simulink model "diagrama_de_bloques"  (R2017b)
settings: Solver=FixedStepDiscrete  StartTime=0.0  StopTime=erle.T_simulacion  FixedStep=erle.Tm  RelTol=1e-3
undefined symbols (not defined in the file or in its folder): erle
settings Model: Creator=javi  LastModifiedBy=javi
settings DataIOCC: SaveFormat=Array

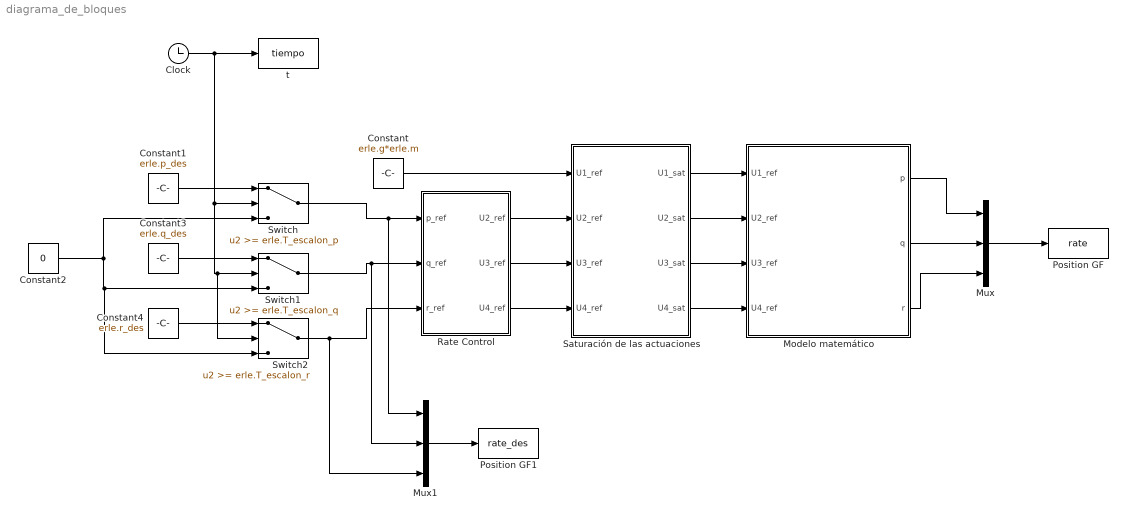
== system diagrama_de_bloques ==
  Clock : Clock
  Constant : Constant  Value=erle.g*erle.m
  Constant1 : Constant  Value=erle.p_des
  Constant2 : Constant  Value=0
  Constant3 : Constant  Value=erle.q_des
  Constant4 : Constant  Value=erle.r_des
  Modelo matemático : Subsystem
  Mux : Mux  Inputs=3
  Mux1 : Mux  Inputs=3
  Position GF : ToWorkspace  VariableName=rate  SampleTime=erle.Tm
  Position GF1 : ToWorkspace  VariableName=rate_des  SampleTime=erle.Tm
  Rate Control : Subsystem
  Saturación de las actuaciones : Subsystem
  Switch : Switch  Threshold=erle.T_escalon_p
  Switch1 : Switch  Threshold=erle.T_escalon_q
  Switch2 : Switch  Threshold=erle.T_escalon_r
  "t " : ToWorkspace  VariableName=tiempo  SampleTime=erle.Tm
  wires:
  Rate Control/1(U2_ref) -> Saturación de las actuaciones/2(U2_ref)
  Rate Control/2(U3_ref) -> Saturación de las actuaciones/3(U3_ref)
  Rate Control/3(U4_ref) -> Saturación de las actuaciones/4(U4_ref)
  Saturación de las actuaciones/1(U1_sat) -> Modelo matemático/1(U1_ref)
  Saturación de las actuaciones/2(U2_sat) -> Modelo matemático/2(U2_ref)
  Saturación de las actuaciones/3(U3_sat) -> Modelo matemático/3(U3_ref)
  Saturación de las actuaciones/4(U4_sat) -> Modelo matemático/4(U4_ref)
  Modelo matemático/1(p) -> Mux/1
  Modelo matemático/2(q) -> Mux/2
  Modelo matemático/3(r) -> Mux/3
  Mux/1 -> Position GF/1
  Clock/1 -> Switch2/2, Switch1/2, Switch/2, "t "/1
  Constant/1 -> Saturación de las actuaciones/1(U1_ref)
  Switch/1 -> Mux1/1, Rate Control/1(p_ref)
  Switch1/1 -> Mux1/2, Rate Control/2(q_ref)
  Switch2/1 -> Mux1/3, Rate Control/3(r_ref)
  Constant1/1 -> Switch/1
  Constant3/1 -> Switch1/1
  Constant4/1 -> Switch2/1
  Constant2/1 -> Switch2/3, Switch1/3, Switch/3
  Mux1/1 -> Position GF1/1

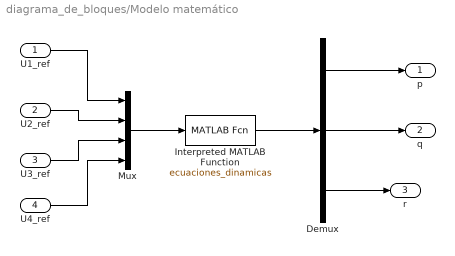
== system diagrama_de_bloques/Modelo matemático ==
  U1_ref : Inport
  U2_ref : Inport  Port=2
  U3_ref : Inport  Port=3
  U4_ref : Inport  Port=4
  Demux : Demux  Outputs=3
  Interpreted MATLAB Function : MATLABFcn  MATLABFcn=ecuaciones_dinamicas  OutputDimensions=3
  Mux : Mux
  p : Outport
  q : Outport  Port=2
  r : Outport  Port=3
  wires:
  U3_ref/1 -> Mux/3
  Mux/1 -> Interpreted MATLAB Function/1
  U2_ref/1 -> Mux/2
  U4_ref/1 -> Mux/4
  U1_ref/1 -> Mux/1
  Interpreted MATLAB Function/1 -> Demux/1
  Demux/1 -> p/1
  Demux/2 -> q/1
  Demux/3 -> r/1

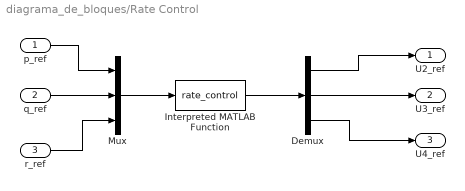
== system diagrama_de_bloques/Rate Control ==
  p_ref : Inport
  q_ref : Inport  Port=2
  r_ref : Inport  Port=3
  Demux : Demux  Outputs=3
  Interpreted MATLAB Function : MATLABFcn  MATLABFcn=rate_control
  Mux : Mux  Inputs=3
  U2_ref : Outport
  U3_ref : Outport  Port=2
  U4_ref : Outport  Port=3
  wires:
  Demux/3 -> U4_ref/1
  Interpreted MATLAB Function/1 -> Demux/1
  Demux/1 -> U2_ref/1
  q_ref/1 -> Mux/2
  Demux/2 -> U3_ref/1
  p_ref/1 -> Mux/1
  r_ref/1 -> Mux/3
  Mux/1 -> Interpreted MATLAB Function/1

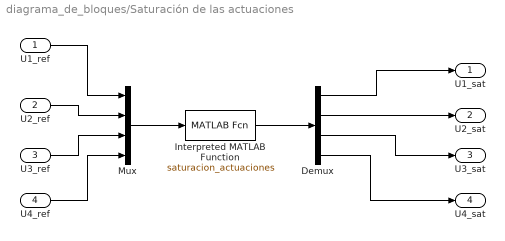
== system diagrama_de_bloques/Saturación de las actuaciones ==
  U1_ref : Inport
  U2_ref : Inport  Port=2
  U3_ref : Inport  Port=3
  U4_ref : Inport  Port=4
  Demux : Demux
  Interpreted MATLAB Function : MATLABFcn  MATLABFcn=saturacion_actuaciones  OutputDimensions=4
  Mux : Mux
  U1_sat : Outport
  U2_sat : Outport  Port=2
  U3_sat : Outport  Port=3
  U4_sat : Outport  Port=4
  wires:
  Demux/1 -> U1_sat/1
  Interpreted MATLAB Function/1 -> Demux/1
  Demux/2 -> U2_sat/1
  U3_ref/1 -> Mux/3
  Demux/3 -> U3_sat/1
  U4_ref/1 -> Mux/4
  U2_ref/1 -> Mux/2
  U1_ref/1 -> Mux/1
  Demux/4 -> U4_sat/1
  Mux/1 -> Interpreted MATLAB Function/1
